simulink model "model_linearised"  (R2025b)
settings: Solver=VariableStepAuto  StartTime=0.0  StopTime=10.0  RelTol=1e-3
undefined symbols (not defined in the file): bm, J, Km, La, motor_func, Ra, Re, Ua_bar, Ue_bar, x1_ini, x2_ini, x3_ini
libraries: simulink x3
settings Model: Creator=adche  LastModifiedBy=adche

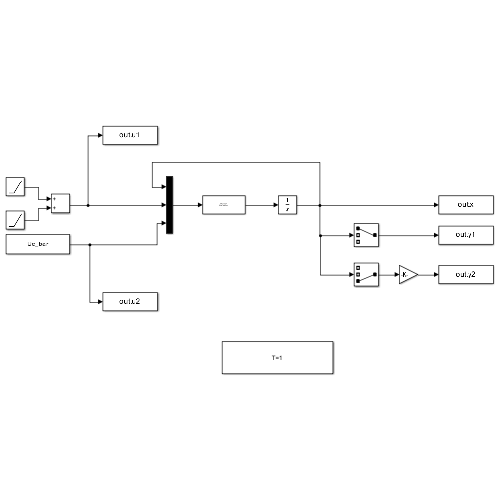
[thumbnail: Simulink's stored preview of the top-level diagram]
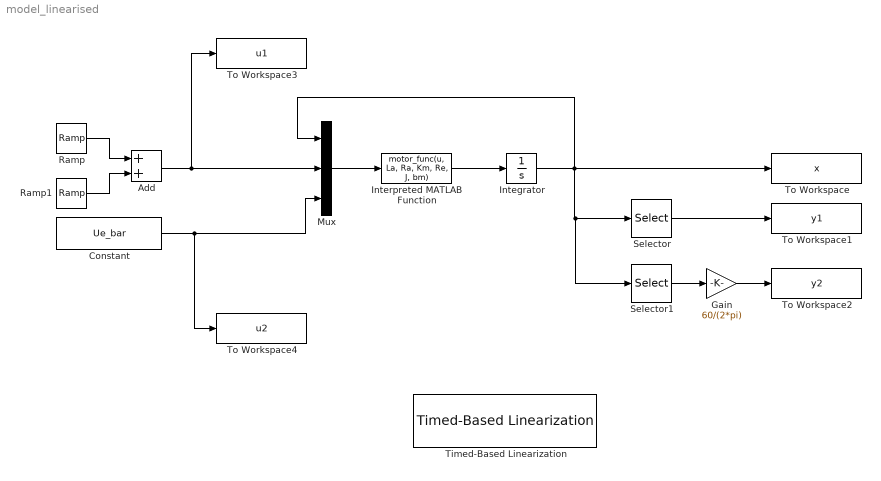
== system model_linearised ==
  Add : Sum
  Constant : Constant  Value=Ue_bar
  Gain : Gain  Gain=60/(2*pi)
  Integrator : Integrator  InitialCondition=[x1_ini x2_ini x3_ini]
  Interpreted MATLAB Function : MATLABFcn  MATLABFcn=motor_func(u, La, Ra, Km, Re, J, bm)
  Mux : Mux  Inputs=3
  Ramp : simulink/Sources/Ramp  slope=Ua_bar/10  start=10  InitialOutput=0
  Ramp1 : simulink/Sources/Ramp  slope=-Ua_bar/10  start=20  InitialOutput=0
  Selector : Selector  InputPortWidth=3  IndexOptions=Index vector (dialog)  Indices=[1]  OutputSizes=1
  Selector1 : Selector  InputPortWidth=3  IndexOptions=Index vector (dialog)  Indices=[3]  OutputSizes=1
  Timed-Based Linearization : simulink/Model-Wide Utilities/Timed-Based Linearization  LinearizationTime=1  SampleTime=0
  To Workspace : ToWorkspace  VariableName=x  SaveFormat=Timeseries  SampleTime=-1
  To Workspace1 : ToWorkspace  VariableName=y1  SaveFormat=Timeseries  SampleTime=-1
  To Workspace2 : ToWorkspace  VariableName=y2  SaveFormat=Timeseries  SampleTime=-1
  To Workspace3 : ToWorkspace  VariableName=u1  SaveFormat=Timeseries  SampleTime=-1
  To Workspace4 : ToWorkspace  VariableName=u2  SaveFormat=Timeseries  SampleTime=-1
  wires:
  Gain/1 -> To Workspace2/1
  Ramp1/1 -> Add/2
  Constant/1 -> To Workspace4/1, Mux/3
  Integrator/1 -> Selector1/1, Selector/1, To Workspace/1, Mux/1
  Selector/1 -> To Workspace1/1
  Interpreted MATLAB Function/1 -> Integrator/1
  Selector1/1 -> Gain/1
  Ramp/1 -> Add/1
  Add/1 -> To Workspace3/1, Mux/2
  Mux/1 -> Interpreted MATLAB Function/1
